simulink model "L1_1"  (Simulink 7.9)
settings: Solver=ode45  StartTime=0.0  StopTime=10.0  RelTol=1e-3
libraries: simulink x1
settings Model: Creator=Павло  LastModifiedBy=Павло

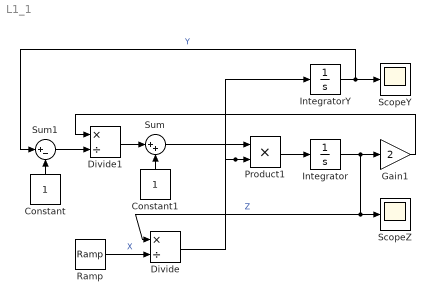
== system L1_1 ==
  Constant : Constant
  Constant1 : Constant
  Divide : Product  Inputs=*/
  Divide1 : Product  Inputs=*/
  Gain1 : Gain  Gain=2
      settings: AttributesFormatString=2
  Integrator : Integrator
  IntegratorY : Integrator
  Product1 : Product  RndMeth=Zero
  Ramp : simulink/Sources/Ramp  slope=2  start=0  X0=1
  ScopeY : Scope
  ScopeZ : Scope
      settings: TickLabels=on  TimeRange=0.9379378758757522  YMin=0.2922020202020199  YMax=0.54820202020202
  Sum : Sum  Inputs=|++
  Sum1 : Sum  Inputs=|+-
  wires:
  Constant/1 -> Sum1/2
  Ramp/1 -> Divide/2  "X"
  Integrator/1 -> Gain1/1, Divide/1, ScopeZ/1  "Z"
  Product1/1 -> Integrator/1
  Constant1/1 -> Sum/2
  Sum/1 -> Product1/1
  Divide/1 -> IntegratorY/1, Product1/2
  Divide1/1 -> Sum/1
  Gain1/1 -> Divide1/1
  IntegratorY/1 -> Sum1/1, ScopeY/1  "Y"
  Sum1/1 -> Divide1/2
